simulink model "POWER_SYSTEM_FULL"  (R2025a)
settings: Solver=ode23t  StartTime=0  StopTime=5  FixedStep=1e-06  MinStep=1e-06  AbsTol=1e-6
model workspace (MAT data in the model file):
  CONTROL_INI : object (value not decoded)
  MODEL_INI : object (value not decoded)
  initialMemoryState = [1.15301991484 1.15301991484 1.15301991484 1.15301991484 0.612188611368 0.612188611368 0.612188611368 0.612188611368 -1.07438763375 -1.07438763375 -1.0821166602 -1.0821166602 ... (40 elements, 40x1)]
symbols that are objects in the model workspace (value not decoded): CONTROL_INI, MODEL_INI
undefined symbols (not defined in the file or in its folder): CONTROL, MODEL, monitorDFIG, pref_mask_vec, qref_mask_vec
(part 2 of 3)

== matlab function POWER_SYSTEM_FULL/DFIG ==
  settings: updateMethod=CONTINUOUS  sampleTime=MODEL_INI.PARAM.SIM_SAMPLING_TIME
  data: STATE input; INPUT input size=4*MODEL_INI.DFIG.PARAM.nDFIG+3; MODEL_IN input Bus: MODEL_Bus; STATE_DERIVATIVE output; OUTPUT output size=10*MODEL_INI.DFIG.PARAM.nDFIG; MODEL output Bus: MODEL_Bus; outSignals output; breaker_status input size=[1,4]; vw_delta input size=[1,4]
function [STATE_DERIVATIVE,OUTPUT,MODEL,outSignals] = DFIG_MODEL(STATE,INPUT,MODEL_IN,breaker_status, vw_delta)

%% COPY MODEL_BUS
MODEL = MODEL_IN;
nDFIG = 4;

%--------------------------------------------------------------------------
%% PARAMETERS
%--------------------------------------------------------------------------
% Rated frequency
f0 = MODEL.BASE.f0;
w0 = 2*pi*f0;
%--------------------------------------------------------------------------
% Induction machine parameters
%--------------------------------------------------------------------------
% Magnetizing reactance
Lm = MODEL.DFIG.PARAM.Lm_pu;
% Stator and rotor leakage reactances
ls = MODEL.DFIG.PARAM.Lsig_s_pu;
lr = MODEL.DFIG.PARAM.Lsig_r_pu;
% Stator and rotor resistances
Rs = MODEL.DFIG.PARAM.Rs_pu;
Rr = MODEL.DFIG.PARAM.Rr_pu;
% Auxiliar electric parameters
Ls = Lm + ls;
Lr = Lm + lr;
sg = 1 - Lm.^2./Ls./Lr;
%--------------------------------------------------------------------------
% DC-link
%--------------------------------------------------------------------------
% DC-link capacitor
Cdc = MODEL.DFIG.PARAM.Cdc_pu;
%--------------------------------------------------------------------------
% DC-LINK BRAKING CHOPPER  (Reviewer 1, point 2 -- fault ride-through)
%--------------------------------------------------------------------------
% LOCAL CONSTANTS, deliberately NOT read from the MODEL bus: adding a bus
% field would change the bus definition and force bus regeneration, which
% project_config.json classifies as a dangerous structural modification.
% Same convention as the converter current limiter in the CONTROL chart.
%
% WHY IT EXISTS -- measured, not speculative.  With the converter current
% limiter armed, a deep sag drove Vdc to 1.52 pu.  Without a chopper the
% DFIG has no way to dump rotor power when the GSC cannot export it: during
% a sag the terminal voltage collapses, the GSC's exportable power falls to
% ~0, and the rotor keeps delivering into the DC link.  No fault-ride-through
% claim is credible without it.
%
% CHOP_EN  Master enable.  0 = DISABLED (default), 1 = ARMED.  With
%          CHOP_EN = 0 the dissipation term is multiplied out to exactly
%          zero, so the model reproduces the no-chopper behaviour bit-for-bit
%          and every published result is unchanged.
CHOP_EN = 0;
%
% VDC_CHOP_ON / VDC_CHOP_OFF  Engage / release thresholds [pu on
%          MODEL.DFIG.BASE.Udc_base = 1200 V], against Vdc_ref = 1.0 pu.
%            VDC_CHOP_OFF = 1.05 pu = 1260 V  -- fully released below this.
%            VDC_CHOP_ON  = 1.10 pu = 1320 V  -- engage threshold.
%          1.05 pu leaves 5 % headroom above nominal so that normal operation
%          and normal transients never reach the chopper.  1.10 pu engages
%          well below the ~1.15-1.20 pu region where DC-link over-voltage
%          protection would trip a real converter, so the chopper acts BEFORE
%          the trip rather than instead of it.  The 0.05 pu band is the
%          conventional "few percent" hysteresis width.
%
%          THEIR ROLE IN THE DUTY REGULATOR (see K_CHOP below): VDC_CHOP_ON is
%          the REGULATION SETPOINT the duty drives Vdc toward, and the band
%          VDC_CHOP_ON - VDC_CHOP_OFF = 0.05 pu is the regulator's DROOP, i.e.
%          the reciprocal of its proportional gain.  Both constants keep their
%          numerical values and their engineering meaning; what changed is that
%          the chopper now MODULATES around VDC_CHOP_ON instead of being pinned
%          at full duty from VDC_CHOP_ON upwards.
VDC_CHOP_ON  = 1.10;
VDC_CHOP_OFF = 1.05;
%
% R_CHOP   Braking-resistor value [pu on MODEL.DFIG.BASE.Zdc_base =
%          Udc_base^2/Sb = 1200^2/2.1034e6 = 0.684605 ohm].
%
%          SIZING -- absorb the rotor power at the worst condition:
%            1. Measured at the optimisation operating point (from the stored
%               LIN_MODEL_VI_OPT): wr = 1.1575, so slip s = 1 - wr = -0.1575
%               (super-synchronous), stator power Ps = 0.849 pu, giving
%               rotor power |Pr| = |s|*Ps = 0.1337 pu flowing OUT of the
%               rotor and into the DC link.
%            2. Worst case: during the sag the rotor ACCELERATES (the slow
%               rotor-speed runaway already characterised), so |s| grows from
%               0.1575 toward the converter's design slip limit of 0.30.  At
%               |s| = 0.30 with stator power at rated 1.0 pu, |Pr| = 0.30 pu.
%            3. The GSC cannot help: at 0.05 pu retained voltage, clamped to
%               its 0.34 pu current rating, its exportable power is only
%               0.34*0.05 = 0.017 pu ~ 0.  So essentially ALL of Pr must be
%               dissipated by the chopper.
%            4. Design margin x1.67 over 0.30 pu to cover the rotor-current
%               surge at fault inception, where the instantaneous P_RSC is
%               well above the steady-state rotor power:
%                     P_chop_rated = 0.50 pu  (= 1.05 MW at Sb = 2.1034 MVA)
%            5. The resistor was sized so that the ORIGINAL on/off law reached
%               full dissipation at Vdc = VDC_CHOP_ON:
%                     R_CHOP = VDC_CHOP_ON^2 / P_chop_rated
%                            = 1.10^2 / 0.50 = 1.21 / 0.50 = 2.42 pu
%               Physical value: 2.42 * 0.684605 = 1.6567 ohm.
%          CROSS-CHECK in SI: at 1320 V across 1.6567 ohm the resistor
%          dissipates 1320^2/1.6567 = 1.0517 MW = 0.500 pu of 2.1034 MVA.
%
%          R_CHOP IS UNCHANGED BY THE MOVE TO A REGULATING DUTY.  It is the
%          resistor's MAXIMUM CAPABILITY, reached only at duty 1; what the duty
%          regulator changes is HOW MUCH OF THAT CAPABILITY IS USED.  Under the
%          regulator (see K_CHOP) duty 1 is reached at 1.15 pu rather than at
%          1.10 pu, where the same resistor dissipates 1.15^2/2.42 = 0.5465 pu
%          -- a 9.3 % increase in peak capability, which is inside the x1.67
%          design margin of step 4 and does not re-open the sizing.
R_CHOP = 2.42;
%
% K_CHOP   Proportional gain of the chopper DUTY REGULATOR
%          [pu duty per pu DC-link voltage].
%
%          WHY THE ON/OFF LAW WAS WRONG -- MEASURED, not speculative.  The
%          first implementation set the duty from the position of Vdc inside
%          the threshold band and SATURATED it at 1 from VDC_CHOP_ON upwards.
%          That makes the chopper a BANG-BANG FULL-POWER DRAIN the moment it is
%          armed.  In the deep-sag run (retained 0.05 pu, SCR = 1, P = 0.8) it
%          dissipated Vdc^2/R_CHOP = 1.23^2/2.42 = 0.625 pu at Vdc = 1.23 pu
%          against an actual DC-link surplus of order 0.1-0.2 pu, and over the
%          peak-to-zero window its time-weighted mean P_CHOP = +0.2885 pu was
%          the LARGEST drain term in the balance -- larger than the GSC export.
%          The chopper installed to protect the DC link was a material
%          contributor to the collapse it was meant to prevent, and Vdc went on
%          to reverse sign to -0.6123 pu.
%
%          WHY IT WAS THE WRONG AVERAGE.  A hysteretic chopper does not hold
%          its IGBT on: it CYCLES it, and the MEAN duty over a switching period
%          is whatever the DC-link power balance demands -- it is not a
%          function of where Vdc happens to sit.  In an AVERAGED converter
%          model Vdc is a slow state, not a fast carrier, so the faithful
%          average of that cycling is a REGULATOR: a duty that closes a loop
%          around Vdc and therefore dissipates the SURPLUS, which is exactly
%          what the switching hardware achieves.  A static band-position ->
%          duty map is not the average of a hysteretic chopper; it is the
%          average of a chopper whose IGBT is stuck on.
%
%          THE LAW -- proportional on the over-voltage, referenced to the
%          ENGAGE threshold, saturated to [0,1] and STILL PURELY ALGEBRAIC
%          (no new states, no bus fields):
%                 d_chop = sat( K_CHOP*(Vdc - VDC_CHOP_ON), 0, 1 )
%
%          THE GAIN, and why this value:
%                 K_CHOP = 1/(VDC_CHOP_ON - VDC_CHOP_OFF) = 1/0.05 = 20
%          It is the reciprocal of the EXISTING threshold band, so no new
%          constant is introduced and the two thresholds keep exact meanings
%          (setpoint and droop).  Three consequences, and they are the
%          justification:
%            1. STEADY-STATE ACCURACY.  The droop is 1/K_CHOP = 0.05 pu, so for
%               any surplus within the resistor's capability the chopper holds
%               Vdc inside [1.10, 1.15] pu and the dissipated power settles at
%               the SURPLUS, not at the rating.  Worked against the measured
%               number above: at a 0.12 pu surplus the loop settles at
%               d = 0.12*2.42/1.11^2 = 0.236, burning 0.12 pu -- not 0.625 pu.
%            2. SOLVER STIFFNESS -- MEASURED, NOT ASSUMED.  A slope of 0 -> 1
%               over 0.05 pu is EXACTLY the slope the previous implementation
%               already carried, only shifted up by one band.  The closed-loop
%               DC-link mode it creates,
%                  lambda = -(w0/Cdc)*K_CHOP*(2*Vdc - VDC_CHOP_ON)/R_CHOP
%                         ~ -5.9e3 rad/s   (tau ~ 0.17 ms at Vdc ~ 1.10),
%               is therefore the SAME mode that the 50 % and the 20 % sag cases
%               already integrated to completion under ode23t with MaxStep 1e-3
%               and MinStep 1e-6.  This change introduces NO new fast mode.  A
%               stiffer gain (K_CHOP = 100 would hold Vdc within 1 %) was
%               rejected for exactly that reason: it would put a 34 us mode
%               into a model that has already been observed to fail Newton
%               convergence at hmin in this operating region.
%            3. SATURATION POINT.  Full duty falls at VDC_CHOP_ON + 1/K_CHOP =
%               1.15 pu -- the bottom of the 1.15-1.20 pu band where a real
%               converter's DC-link over-voltage protection trips.  So the
%               resistor reaches its rated dissipation exactly where a real
%               machine would be about to trip, and modulates below it.  This
%               is the same "act BEFORE the trip" intent already recorded for
%               the thresholds, now expressed in the duty rather than in R.
%
%          WHAT THIS DOES NOT CLAIM.  Above 1.15 pu the duty IS 1 and the
%          resistor DOES dissipate its full capability.  That is not a
%          modelling artefact -- a real hysteretic chopper at 1.23 pu is also
%          hard on, continuously.  What is fixed here is the pinning of the
%          duty at 1 across the WHOLE armed range; what no duty law can fix is
%          an over-sized resistor, and R_CHOP is deliberately left at its
%          original value so that this change is the duty and nothing else.
K_CHOP = 1./(VDC_CHOP_ON - VDC_CHOP_OFF);
%--------------------------------------------------------------------------
% DC-LINK DIVISION GUARD -- NUMERICAL, UNCONDITIONAL
%--------------------------------------------------------------------------
% VDC_FLOOR  Denominator floor for the DC-link current map  idc = Pdc/Vdc.
%          This is a NUMERICAL GUARD, NOT a control or protection feature, so
%          it is DELIBERATELY NOT gated on CHOP_EN or on any other switch: an
%          unguarded division belongs in no version of the model.  It is the
%          exact analogue of VS_FLOOR in the CONTROL chart, one chart over.
%
%          WHY IT EXISTS -- measured, not speculative.  In a deep sag (0.05 pu
%          retained) the DC link does NOT over-charge, it DRAINS: the terminal
%          voltage collapses, so the GSC can import at most 0.34*0.05 = 0.017
%          pu while the RSC keeps drawing from the capacitor.  Vdc was measured
%          falling through 0.3219 pu at the instant the solver died with
%          NewtonIterationFailure at hmin, 8.68 ms after inception.  As
%          Vdc -> 0 both the map idc = Pdc/Vdc and its Jacobian entry
%          d(idc)/d(Vdc) = -Pdc/Vdc^2 blow up, and nothing downstream can
%          rescue it: min/max propagate Inf and NaN rather than clamping them.
%          The braking chopper cannot help -- it only acts above
%          VDC_CHOP_OFF = 1.05 pu and addresses the OPPOSITE excursion.
%
%          VALUE: 0.50 pu = 600 V on Udc_base = 1200 V.  The justification is
%          that at and below this DC voltage the RSC has already lost control
%          authority, so the AVERAGED converter model -- whose core assumption
%          is that vr and vg are imposed EXACTLY as commanded -- is outside its
%          validity range regardless of what the division does:
%            - With SVPWM a two-level bridge synthesises at most Vdc/sqrt(2)
%              of line-to-line RMS AC voltage.  At Vdc = 0.50 pu = 600 V that
%              is 424.3 V, i.e. 424.3/2070 = 0.205 pu on the rotor base
%              (Ur_open_rotor_V = 2070 V = 3 pu of Ub = 690 V).
%            - The rotor back-EMF ALONE is |s|*|Fs|*Lm/Ls = 0.1575*1*
%              2.0033/2.0731 = 0.152 pu at the pre-fault slip, and it GROWS as
%              the rotor accelerates during the fault.  So at 0.50 pu the RSC
%              retains under 35 % margin over the back-EMF BEFORE the resistive
%              and di/dt terms -- it can no longer impose the commanded rotor
%              voltage, and the model has stopped describing the machine.
%            - For scale, the DC link is sized for the full +-0.30 design slip:
%              |vr| = 0.30*2070 = 621 V needs Vdc >= sqrt(2)*621 = 878 V =
%              0.73 pu, against the 1.0 pu nominal.
%
%          The floor is INACTIVE in every legitimate transient measured.  The
%          deepest Vdc excursion in any run that integrates to completion is
%          0.6679 pu (50 % sag, 150 ms, limiter and chopper armed), 25 % above
%          the floor; the 20 % / 500 ms case reaches 0.6892 pu.  At both
%          linearisation operating points Vdc = 1.0 pu exactly, so
%          Vdc_safe == Vdc and the guard is invisible to the small-signal
%          model.  That is verified, not asserted, by the zero-difference
%          regression at all four switch combinations.
VDC_FLOOR = 0.50;
%--------------------------------------------------------------------------
% DC-LINK DIODE CLAMP -- PHYSICS, UNCONDITIONAL, NO NEW STATES
%--------------------------------------------------------------------------
% VDC_DIODE / VDC_DIODE_BAND  One-sided LOWER clamp on the DC-link voltage,
%          enforcing in the averaged model what the converters' ANTI-PARALLEL
%          DIODES enforce in hardware: the DC link cannot be discharged
%          through zero.  Measured motivation -- in a deep sag the stator
%          power collapses, there is no slip power left to trap, P_RSC FLIPS
%          POSITIVE (it pushes INTO the rotor to hold |ir| at the limit
%          against collapsed flux) while the GSC still exports, and the link
%          drains to Vdc = -0.5825 pu.  A negative DC-link voltage is not a
%          small error, it is impossible: the diodes clamp it.
%
%          THIS IS NOT VDC_FLOOR AND MUST NOT BE CONFLATED WITH IT.  They are
%          different objects doing different jobs and the paper must keep them
%          apart:
%            - VDC_FLOOR = 0.50 pu is a NUMERICAL guard on a DIVISION.  It
%              bounds the DENOMINATOR of idc = Pdc/Vdc so the map and its
%              Jacobian stay finite.  It is a statement about ARITHMETIC.
%              Where it is active the trajectory is an ARTEFACT OF THE GUARD
%              and no quantitative claim may rest on it.
%            - VDC_DIODE is a PHYSICAL constraint on the STATE.  It says a
%              capacitor bridged by anti-parallel diodes cannot reverse
%              polarity.  Where it is active the trajectory is STILL PHYSICS:
%              it is the physics of a link being held up by its own diodes.
%          A run that touches VDC_FLOOR has left the model's validity range;
%          a run that touches VDC_DIODE has not.  Reporting the two as the
%          same event would overstate the model's reach in exactly the way
%          quoting the source voltage instead of the PCC voltage does.
%
%          WHY IT CANNOT BE A max() ON Vdc.  Vdc is STATE 6, not an algebraic
%          quantity.  A max() here would clamp the value the chart READS while
%          the integrator went on driving the true state further negative; the
%          clamp would then silently unlatch on the way back up, and the
%          reported Vdc would no longer be the model's own state.  The
%          physically correct statement is a ONE-SIDED CONSTRAINT ON THE
%          DERIVATIVE: discharge is progressively refused as Vdc approaches
%          the clamp, charge is never impeded.  That is what is implemented at
%          the dVdc assignment below, and it adds NO state and NO bus field.
%
%          VALUE: 0.05 pu = 60 V on Udc_base = 1200 V.  Zero is the strict
%          physical bound; 0.05 pu sits just above it, deliberately.  First,
%          it keeps the state away from the exact zero at which the UNGUARDED
%          map idc = Pdc/Vdc changes sign, so the diode clamp does not lean on
%          VDC_FLOOR to stay finite and the two stay independent -- which is
%          the whole point of separating them.  Second, a real diode clamp
%          holds the link at the RECTIFIED PEAK of the AC side, which is well
%          above zero; 0.05 pu is a deliberately conservative stand-in for
%          that bound, not an attempt to model it.
%
%          SCOPE, STATED PLAINLY: the entire clamp lives at 0.15 pu and below,
%          i.e. wholly INSIDE the region VDC_FLOOR has already declared
%          numerically guarded.  It can therefore only ever rescue criterion
%          (a) (Vdc > 0) and CANNOT move criterion (b) (Vdc >= VDC_FLOOR).
%          It is not intended to.  Moving (b) is the RSC blocking's job, one
%          chart over -- the clamp bounds the consequence, the blocking
%          removes the cause.
VDC_DIODE = 0.05;
% VDC_DIODE_BAND  Blend width [pu] of the clamp gate.
%          A HARD kink at the clamp would be worse than the singularity it
%          replaces: it makes dVdc discontinuous in a state and forces ode23t
%          to chatter its Newton iteration across the crossing.  The gate is
%          therefore a SMOOTHSTEP s^2*(3-2s) over [VDC_DIODE, VDC_DIODE+BAND],
%          which is C1 -- ZERO SLOPE AT BOTH ENDS.
%            - Zero slope at the UPPER end is what makes the clamp exactly
%              invisible to the linearisation.  The gate is not merely EQUAL
%              to 1 at the operating point (Vdc = 1.0 pu, 8.5 band-widths
%              above the top of the band); its derivative with respect to Vdc
%              is also exactly 0 there, so no numericalpert step of order
%              1e-5 can see it.
%            - Zero slope at the LOWER end gives a soft landing: the approach
%              to the clamp decelerates quadratically rather than stopping in
%              a corner, so the solver is not asked to resolve an impact.
VDC_DIODE_BAND = 0.10;
%--------------------------------------------------------------------------
% GSC filter
%--------------------------------------------------------------------------
% GSC filter resistance
Rfg = MODEL.DFIG.PARAM.Rfgsc_pu;
% GSC filter reactance
Lfg = MODEL.DFIG.PARAM.Lfgsc_pu;
%--------------------------------------------------------------------------
% Transformer
%--------------------------------------------------------------------------
% Transformer resistance
Rt = MODEL.DFIG.PARAM.Rt_pu;
% Transformer inductance
Lt = MODEL.DFIG.PARAM.Lt_pu;
%--------------------------------------------------------------------------
% Mechanical model (2 masses)
%--------------------------------------------------------------------------
Ht = MODEL.DFIG.PARAM.Ht_pu;
Dt = MODEL.DFIG.PARAM.Dt_pu;
Hg = MODEL.DFIG.PARAM.Hg_pu;
Dg = MODEL.DFIG.PARAM.Dg_pu;
Dtg = MODEL.DFIG.PARAM.Dtg_pu;
Ktg = MODEL.DFIG.PARAM.Ktg_pu;
%--------------------------------------------------------------------------
% Turbine
%--------------------------------------------------------------------------
% Turbine data
turbineData = MODEL.DFIG.PARAM.turbineData;

%--------------------------------------------------------------------------
% State-space representation with transformer
%--------------------------------------------------------------------------
% it = -(ig + is)
% 1/w0*dFs + 1j*w*Fs         = vs - Rs.*is;       % is flows into the IM 
% 1/w0*dFr + 1j*(w - wr).*Fr = vr - Rr.*ir;       % ir flows into the IM
% 1/w0*dFg + 1j*w*Fg         = vs - vg - Rfg.*ig; % ig flows into the GSC
% 1/w0*dFt + 1j*w*Ft         = vs - vp - Rt.*it;  % it flows into the PCC
%--------------------------------------------------------------------------
% Fst = Fs - Ft
% Fgt = Fg - Ft
%--------------------------------------------------------------------------
% 1./w0.*dFst + 1j*w.*Fst = vp + Rt.*it - Rs.*is;
% 1./w0.*dFgt + 1j*w.*Fgt = vp + Rt.*it - vg - Rfg.*ig;
%--------------------------------------------------------------------------
% 1./w0.*dFst + 1j*w.*Fst = vp - (Rs + Rt).*is - Rt.*ig;
% 1./w0.*dFgt + 1j*w.*Fgt = vp - vg - Rt.*is - (Rfg + Rt).*ig;
%--------------------------------------------------------------------------
% Fg = Lfg.*ig
% Ft = Lt.*it
% Fs = Ls.*is + Lm.*ir
% Fr = Lm.*is + Lr.*ir
%--------------------------------------------------------------------------
% Fgt = Lfg.*ig - Lt.*it = (Lfg + Lt).*ig + Lt.*is
% Fst = Ls.*is + Lm.*ir - Lt.*it = (Ls + Lt).*is + Lt.*ig + Lm.*ir
% Lm.*ir = Lm./Lr.*(Fr - Lm.*is)
% Fst - Lm./Lr.*Fr = (sg.*Ls + Lt).*is + Lt.*ig
%--------------------------------------------------------------------------
% [Fgt ; Fst - Lm./Lr.*Fr] = [Lfg+Lt   Lt ; Lt  sg*Ls+Lt]*[ig ; is]
% [ig ; is] = inv([Lfg+Lt   Lt ; Lt  sg*Ls+Lt])*[Fgt ; Fst - Lm./Lr.*Fr]
% |Lfg+Lt   Lt ; Lt  sg*Ls+Lt| = (Lfg+Lt)*(sg*Ls+Lt) - Lt^2 = 
%                             = sg*Ls*Lfg + (Lfg+sg*Ls)*Lt
% inv([Lfg+Lt   Lt ; Lt  sg*Ls+Lt]) = [sg*Ls+Lt -Lt ; -Lt Lfg+Lt]/(sg*Ls*Lfg + (Lfg+sg*Ls)*Lt)
%--------------------------------------------------------------------------
% ig = ((sg.*Ls+Lt).*Fgt - Lt.*(Fst - Lm./Lr.*Fr))./(sg.*Ls.*Lfg + (Lfg+sg*Ls).*Lt)
% is = (-Lt.*Fgt  + (Lfg + Lt).*(Fst - Lm./Lr.*Fr))./(sg.*Ls.*Lfg + (Lfg+sg*Ls).*Lt)
% it = -(ig + is)
% Fs = Ls.*is + Lm.*ir = Ls.*is + Lm./Lr.*(Fr - Lm.*is) = sg.*Ls.*is + Lm./Lr.*Fr;
% Ft = Fs - Fst;
% Fg = Fgt + Ft;
% ir = 1./Lm.*(Fs - Ls.*is)
% dis = (-Lt.*Fgt  + (Lfg + Lt).*(dFst - Lm./Lr.*dFr))./(sg.*Ls.*Lfg + (Lfg+sg*Ls).*Lt)
% 1./w0*dFs = sg.*Ls.*dis + Lm./Lr.*dFr
% vs = 1/w0*dFs + 1j*w*Fs + Rs*is
%--------------------------------------------------------------------------

%--------------------------------------------------------------------------
%% STATE
%--------------------------------------------------------------------------
% Stator flux - Transformer flux
%--------------------------------------------------------------------------
Fst_r = STATE(1,:);
Fst_i = STATE(2,:);
Fst = Fst_r + 1j*Fst_i;
%--------------------------------------------------------------------------
% Rotor flux
%--------------------------------------------------------------------------
Fr_r = STATE(3,:);
Fr_i = STATE(4,:);
Fr = Fr_r + 1j*Fr_i;
%--------------------------------------------------------------------------
% Rotor speed
%--------------------------------------------------------------------------
wr = STATE(5,:);
%--------------------------------------------------------------------------
% DC-Link voltage
%--------------------------------------------------------------------------
Vdc = STATE(6,:);
%--------------------------------------------------------------------------
% GSC flux - transformer flux
%--------------------------------------------------------------------------
Fgt_r = STATE(7,:);
Fgt_i = STATE(8,:);
Fgt = Fgt_r + 1j*Fgt_i;
%--------------------------------------------------------------------------
% Mechanical shaft
%--------------------------------------------------------------------------
wt = STATE(9,:);
Ttg = STATE(10,:);

%--------------------------------------------------------------------------
%% INPUT
%--------------------------------------------------------------------------
% INPUT = [vrr ; vri ; vgr ; vgi ; w ; vpr ; vpi]
nDFIG = 4;
vrr = INPUT(0*nDFIG + (1:nDFIG))';
vri = INPUT(1*nDFIG + (1:nDFIG))';
vgr = INPUT(2*nDFIG + (1:nDFIG))';
vgi = INPUT(3*nDFIG + (1:nDFIG))';
w   = INPUT(4*nDFIG + 1);
vpr = INPUT(4*nDFIG + 2);
vpi = INPUT(4*nDFIG + 3);
%--------------------------------------------------------------------------
% RSC voltage
%--------------------------------------------------------------------------
MODEL.DFIG.INPUT.vRSC_r = vrr;
MODEL.DFIG.INPUT.vRSC_i = vri;
vr = vrr + 1j*vri;
%--------------------------------------------------------------------------
% GSC voltage
%--------------------------------------------------------------------------
MODEL.DFIG.INPUT.vGSC_r = vgr;
MODEL.DFIG.INPUT.vGSC_i = vgi; 
vg = vgr + 1j*vgi;
%--------------------------------------------------------------------------
% PCC voltage
%--------------------------------------------------------------------------
MODEL.DFIG.INPUT.vPCC_r = vpr*ones(1,nDFIG);
MODEL.DFIG.INPUT.vPCC_i = vpi*ones(1,nDFIG); 
vp = vpr + 1j*vpi;
%--------------------------------------------------------------------------
% Grid frequency [pu]
%--------------------------------------------------------------------------
MODEL.GRID.OUTPUT.f_pu = w;
%--------------------------------------------------------------------------
% Wind speed [m/s]
%--------------------------------------------------------------------------
windSpeed = MODEL.DFIG.INPUT.windSpeed + vw_delta;
%% vw_delta [1x4]: additive wind speed perturbation (m/s), zeros at op point
%--------------------------------------------------------------------------
% Turbine pitch [deg]
%--------------------------------------------------------------------------
pitch = MODEL.DFIG.INPUT.turbinePitch;


%--------------------------------------------------------------------------
%% ELECTRIC VARIABLES
%--------------------------------------------------------------------------
% Stator current
%--------------------------------------------------------------------------
is = (-Lt.*Fgt + (Lfg + Lt).*(Fst - Lm./Lr.*Fr))./(sg.*Ls.*Lfg + (Lfg+sg.*Ls).*Lt);
isr = real(is);
isi = imag(is);
%--------------------------------------------------------------------------
% Fluxes
%--------------------------------------------------------------------------
Fs = sg.*Ls.*is + Lm./Lr.*Fr;
Ft = Fs - Fst;
Fg = Fgt + Ft;
%--------------------------------------------------------------------------
% Rotor current
%--------------------------------------------------------------------------
ir = 1./Lm.*(Fs - Ls.*is);
irr = real(ir);
iri = imag(ir);
%--------------------------------------------------------------------------
% Grid current
%--------------------------------------------------------------------------
ig = 1./Lfg.*Fg; 
igr = real(ig); 
igi = imag(ig);
%--------------------------------------------------------------------------
% Transformer current
%--------------------------------------------------------------------------
it = 1./Lt.*Ft; 
itr = real(it); 
iti = imag(it);
%--------------------------------------------------------------------------
% Electric torque (motor torque)
%--------------------------------------------------------------------------
% Te = imag(is*conj(Fs))/sqrt(3)
% Fs = Ls*is + Lm*ir
% Te = imag(is*conj(Ls*is + Lm*ir))/sqrt(3) = Lm*imag(is*conj(ir))/sqrt(3)
Te = Lm.*imag(is.*conj(ir))/sqrt(3);
%--------------------------------------------------------------------------
% Power computation in DC link
%--------------------------------------------------------------------------
P_GSC = real(vg.*conj(ig))/sqrt(3);
P_RSC = real(vr.*conj(ir))/sqrt(3);
Pdc = P_GSC - P_RSC;
%--------------------------------------------------------------------------
% DC-link braking chopper -- CONDITIONAL DISSIPATION, PURELY ALGEBRAIC
%--------------------------------------------------------------------------
% Sign convention check: Pdc = P_GSC - P_RSC charges the capacitor, since
% dVdc = w0*idc/Cdc with idc = Pdc/Vdc.  Super-synchronously P_RSC < 0 (the
% rotor DELIVERS), and during a sag P_GSC -> 0 while P_RSC stays negative, so
% Pdc > 0 and Vdc rises.  The chopper therefore SUBTRACTS from Pdc.
%
% d_chop is the chopper DUTY CYCLE: the AVERAGED-MODEL representation of a
% hysteresis-cycled chopper, written as a PROPORTIONAL REGULATOR on the
% DC-link over-voltage.  A true two-valued relay with engage/release memory is
% by definition STATEFUL and the constraint here is NO NEW STATES; but the
% averaged duty is not merely a workaround for that constraint, it is the
% CORRECT representation, because the quantity a real chopper's switching
% produces on the time scale this model resolves IS a mean duty.
%
% The mean duty of a hysteresis-cycled IGBT is set by the DC-LINK POWER
% BALANCE -- the chopper cycles at whatever ratio dissipates the instantaneous
% surplus and thereby holds Vdc at its threshold.  It is NOT a static function
% of where Vdc sits.  Mapping band position directly onto duty (the previous
% implementation) pins the duty at 1 the moment Vdc leaves the band upwards,
% i.e. it averages a chopper whose IGBT is STUCK ON, and it dumps the
% resistor's full capability whenever armed rather than the surplus.  That was
% measured to be the largest single drain term in the deep-sag DC-link
% collapse (see the K_CHOP block above for the numbers).
%
% The regulator form fixes exactly that: VDC_CHOP_ON is the SETPOINT the loop
% drives Vdc toward, K_CHOP = 1/(VDC_CHOP_ON - VDC_CHOP_OFF) is the droop, and
% the saturation to [0,1] is the physical duty limit.  It is still continuous,
% so it does not chatter the variable-step solver the way a bare relay would,
% and it is still purely algebraic.
d_chop = min(max(K_CHOP.*(Vdc - VDC_CHOP_ON),0),1);
% Dissipated power [pu].  Identically 0 when CHOP_EN = 0, and ALSO identically
% 0 whenever Vdc <= VDC_CHOP_ON regardless of CHOP_EN -- which is why the
% linearisation at the operating point (Vdc = 1.0 pu) is unaffected in both
% switch states: the clamp is FLAT there, so the term and its derivative with
% respect to every state are exactly zero.  The margin from the operating
% point to the start of the ramp is now 0.10 pu rather than 0.05 pu, i.e.
% TWICE the previous distance, against a numericalpert step of order 1e-5.
P_CHOP = CHOP_EN .* d_chop .* Vdc.^2 ./ R_CHOP;
Pdc = Pdc - P_CHOP;
%--------------------------------------------------------------------------
% Current in DC link
%--------------------------------------------------------------------------
% Guarded denominator -- see VDC_FLOOR above.  A single unconditional max() is
% sufficient and is NOT gated on any switch.  It also fixes the SIGN: an
% unguarded 1/Vdc flips sign if a solver trial iterate drives Vdc through zero,
% which no Newton iteration can recover from.  Below the floor the map is flat
% in Vdc, so the Jacobian entry -Pdc/Vdc^2 is replaced by exactly 0 instead of
% diverging.  Vdc itself, not Vdc_safe, is what leaves the chart as OUTPUT and
% feeds the chopper duty and the CONTROL chart, so the guard changes the
% DERIVATIVE map only and never falsifies a reported quantity.
Vdc_safe = max(Vdc, VDC_FLOOR);
idc = Pdc./Vdc_safe;

%--------------------------------------------------------------------------
%% MECHANICAL VARIABLES
%--------------------------------------------------------------------------
% Turbine mechanical power
%--------------------------------------------------------------------------
% Mechanical power = 1/2*Cp(Lambda,Pitch)*ro*pi*R^2*windSpeed^3
Pm = WIND_TURBINE_OP(pitch,windSpeed,wt,turbineData);
Pm = Pm.*(Pm>0);
%--------------------------------------------------------------------------
% Turbine mechanical torque
%--------------------------------------------------------------------------
Tm = Pm./wt;

%--------------------------------------------------------------------------
%% STATE DERIVATIVE
%--------------------------------------------------------------------------
% Stator - Transformer Flux 
%--------------------------------------------------------------------------
% 1./w0.*dFst + 1j*w.*Fst = vp - (Rs + Rt).*is - Rt.*ig;
dFst = w0.*(vp - Rt.*ig - (Rt + Rs).*is - 1j.*w.*Fst);
dFst_r = real(dFst); 
dFst_i = imag(dFst);
%--------------------------------------------------------------------------
% Rotor Flux
%--------------------------------------------------------------------------
dFr = w0.*(vr - Rr.*ir - 1j.*(w - wr).*Fr);
dFr_r = real(dFr); 
dFr_i = imag(dFr);
%--------------------------------------------------------------------------
% DC-Link voltage
%--------------------------------------------------------------------------
% DIODE CLAMP -- one-sided constraint on the DERIVATIVE (see VDC_DIODE above).
% Charging is never impeded; discharging is faded out as Vdc approaches the
% clamp level.  The split
%       dVdc = max(dVdc_raw,0) + g.*min(dVdc_raw,0)
% is an EXACT IDENTITY when g = 1, because max(x,0) + min(x,0) == x for every
% x -- in floating point as well as in algebra, since one term is always
% exactly x and the other exactly 0.  Above the band the derivative is
% therefore bit-for-bit the unclamped one, which is why the small-signal
% regression stays EXACTLY zero rather than merely small.
dVdc_raw = w0.*idc./Cdc;
s_diode  = min(max((Vdc - VDC_DIODE)./VDC_DIODE_BAND, 0), 1);
g_diode  = s_diode.^2.*(3 - 2.*s_diode);
dVdc     = max(dVdc_raw,0) + g_diode.*min(dVdc_raw,0);
%--------------------------------------------------------------------------
% GSC - Transformer Flux
%--------------------------------------------------------------------------
% 1./w0.*dFgt + 1j*w.*Fgt = vp - vg - Rt.*is - (Rfg + Rt).*ig;
dFgt = w0.*(vp - vg - Rt.*is - (Rt + Rfg).*ig - 1j*w.*Fgt);
dFgt_r = real(dFgt); 
dFgt_i = imag(dFgt);
%--------------------------------------------------------------------------
% Turbine and shaft dynamics
%--------------------------------------------------------------------------
dwt = (1/2)./Ht.*(Tm - Dt.*wt - Ttg - Dtg.*(wt-wr));
dTtg = w0*Ktg.*(wt-wr);
% dTtg = Ktg.*(wt-wr);
dwr = (1/2)./Hg.*(Ttg + Te - Dg.*wr + Dtg.*(wt-wr));
%--------------------------------------------------------------------------
% State derivative
%--------------------------------------------------------------------------
STATE_DERIVATIVE = [dFst_r ; dFst_i ; dFr_r ; dFr_i ; dwr ; ....
    dVdc ; dFgt_r ; dFgt_i ; dwt ; dTtg];

%--------------------------------------------------------------------------
% BREAKER LOGIC: freeze states of disconnected generators
%--------------------------------------------------------------------------
STATE_DERIVATIVE = STATE_DERIVATIVE .* breaker_status;

%--------------------------------------------------------------------------
%% OUTPUT AND MEASURED VARIABLES
%--------------------------------------------------------------------------
% Stator voltage
%--------------------------------------------------------------------------
dis = (-Lt.*Fgt  + (Lfg + Lt).*(dFst - Lm./Lr.*dFr))./(sg.*Ls.*Lfg + (Lfg+sg.*Ls).*Lt);
dFs = sg.*Ls.*dis + Lm./Lr.*dFr;
vs = 1/w0*dFs + 1j*w*Fs + Rs.*is;
MODEL.DFIG.OUTPUT.vs_r = real(vs);
MODEL.DFIG.OUTPUT.vs_i = imag(vs);
%--------------------------------------------------------------------------
% Currents
%--------------------------------------------------------------------------
% Stator current into the IM
MODEL.DFIG.OUTPUT.is_r = isr;
MODEL.DFIG.OUTPUT.is_i = isi;
% Rotor current into the IM and from the RSC
MODEL.DFIG.OUTPUT.ir_r = irr;
MODEL.DFIG.OUTPUT.ir_i = iri;
% GSC current into the GSC
MODEL.DFIG.OUTPUT.ig_r = igr;
MODEL.DFIG.OUTPUT.ig_i = igi;
% Transformer current into the PCC and from the DFIG
MODEL.DFIG.OUTPUT.it_r = itr;
MODEL.DFIG.OUTPUT.it_i = iti;
%--------------------------------------------------------------------------
% DC-Link Voltage [pu]
%--------------------------------------------------------------------------
MODEL.DFIG.OUTPUT.Vdc = Vdc;
%--------------------------------------------------------------------------
% Converter and DC-Link powers
%--------------------------------------------------------------------------
MODEL.DFIG.OUTPUT.P_GSC = P_GSC;
MODEL.DFIG.OUTPUT.P_RSC = P_RSC;
MODEL.DFIG.OUTPUT.Pdc = Pdc;
%--------------------------------------------------------------------------
% Rotor speed [pu]
%--------------------------------------------------------------------------
MODEL.DFIG.OUTPUT.wr = wr;
%--------------------------------------------------------------------------
% Mechanical power [pu]
%--------------------------------------------------------------------------
MODEL.DFIG.OUTPUT.Pm = Pm;

%--------------------------------------------------------------------------
%% STATE UPDATE
%--------------------------------------------------------------------------
MODEL.DFIG.STATE = STATE;

%--------------------------------------------------------------------------
%% CONNECTIONS WITH THE POWER SYSTEM
%--------------------------------------------------------------------------
%--------------------------------------------------------------------------
% BREAKER LOGIC: zero currents of disconnected generators
%--------------------------------------------------------------------------
itr = itr .* breaker_status;
iti = iti .* breaker_status;
isr = isr .* breaker_status;
isi = isi .* breaker_status;
irr = irr .* breaker_status;
iri = iri .* breaker_status;
igr = igr .* breaker_status;
igi = igi .* breaker_status;

%--------------------------------------------------------------------------
% OUTPUT = [itr ; iti ; isr ; isi ; irr ; iri ; vsr ; vsi ; Vdc ; wr]
%--------------------------------------------------------------------------
OUTPUT = zeros(10*nDFIG,1);
OUTPUT(0*nDFIG + (1:nDFIG)) = itr(:);
OUTPUT(1*nDFIG + (1:nDFIG)) = iti(:);
OUTPUT(2*nDFIG + (1:nDFIG)) = isr(:);
OUTPUT(3*nDFIG + (1:nDFIG)) = isi(:);
OUTPUT(4*nDFIG + (1:nDFIG)) = irr(:);
OUTPUT(5*nDFIG + (1:nDFIG)) = iri(:);
OUTPUT(6*nDFIG + (1:nDFIG)) = real(vs(:));
OUTPUT(7*nDFIG + (1:nDFIG)) = imag(vs(:));
OUTPUT(8*nDFIG + (1:nDFIG)) = Vdc(:);
OUTPUT(9*nDFIG + (1:nDFIG)) = wr(:);

%% Output auxiliary signals
Sdfig = vs.*conj(it)/sqrt(3);
outSignals = [abs(vs(:)),real(Sdfig(:)),imag(Sdfig(:)),Vdc(:)];

return

== matlab function POWER_SYSTEM_FULL/LINE_GRID ==
  settings: updateMethod=CONTINUOUS  sampleTime=MODEL_INI.PARAM.SIM_SAMPLING_TIME
  data: STATE input; INPUT input size=2*MODEL_INI.DFIG.PARAM.nDFIG; MODEL_IN input Bus: MODEL_Bus; STATE_DERIVATIVE output; OUTPUT output size=3; MODEL output Bus: MODEL_Bus; il_r_IN input; il_i_IN input; f_OUT output; Vpcc_OUT output
function [STATE_DERIVATIVE,OUTPUT,MODEL,f_OUT,Vpcc_OUT] = LINE_GRID_MODEL(STATE,INPUT,MODEL_IN,il_r_IN,il_i_IN)

%% COPY MODEL_BUS
MODEL = MODEL_IN;
nDFIG = 4;

%--------------------------------------------------------------------------
%% PARAMETERS
%--------------------------------------------------------------------------
% Rated frequency
%--------------------------------------------------------------------------
f0 = MODEL.BASE.f0;
w0 = 2*pi*f0;

%--------------------------------------------------------------------------
% Grid resistence and inductance
%--------------------------------------------------------------------------
Rg = MODEL.GRID.PARAM.Rg_pu;
Lg = MODEL.GRID.PARAM.Lg_pu;
%--------------------------------------------------------------------------
% Node 1 resistance and capacitance
%--------------------------------------------------------------------------
Rn1 = MODEL.LINE.PARAM.Rn1_pu;
Cn1 = MODEL.LINE.PARAM.Cn1_pu;
%--------------------------------------------------------------------------
% Load perturbation injection node (1=PCC, 2=grid bus)
%--------------------------------------------------------------------------
load_node = MODEL.LINE.PARAM.load_node;
%--------------------------------------------------------------------------
% Speed governor
%--------------------------------------------------------------------------
% Damping (Deq_pu/2) and steady-state droop (2/Deq_pu)
Deq_pu = MODEL.GRID.PARAM.Deq_pu;
% Time constant [s]
Tgov = MODEL.GRID.PARAM.Tgov;
%--------------------------------------------------------------------------
% Turbine (second order: time constants Ttb1 and Ttb2
%--------------------------------------------------------------------------
% [(0.3*7) 1] / [(0.3*7) (0.3+7) 1]
% [(Ttb1*Ttb2) 1] / [(Ttb1*Ttb2) (Ttb1+Ttb2) 1]
% Time constants [s]
Ttb1 = MODEL.GRID.PARAM.Ttb1;
Ttb2 = MODEL.GRID.PARAM.Ttb2;
%--------------------------------------------------------------------------
% Grid inertia [s]
%--------------------------------------------------------------------------
H = MODEL.GRID.PARAM.H;

%--------------------------------------------------------------------------
%% STATE
%--------------------------------------------------------------------------
%--------------------------------------------------------------------------
% Speed governor (first order 1/(Tgov*s+1))
%--------------------------------------------------------------------------
xsg = STATE(1,:);
%--------------------------------------------------------------------------
% Turbine (second order (Ttb1*Ttb2*s + 1)/(Ttb1*Ttb2*s + (Ttb1+Ttb2)*s + 1))
%--------------------------------------------------------------------------
xt1 = STATE(2,:);
xt2 = STATE(3,:);
%--------------------------------------------------------------------------
% Grid frequency [pu]
%--------------------------------------------------------------------------
w = STATE(4,:);
%--------------------------------------------------------------------------
% Line current [pu]
%--------------------------------------------------------------------------
ir = STATE(5,:);
ii = STATE(6,:);
i = ir + 1j*ii;
%--------------------------------------------------------------------------
% Node 1 Voltage [pu]
%--------------------------------------------------------------------------
v1r = STATE(7,:);
v1i = STATE(8,:);
v1 = v1r + 1j*v1i;

%--------------------------------------------------------------------------
%% INPUT
%--------------------------------------------------------------------------
% INPUT = [in1r ; in1i]
in1r = sum(INPUT(0*nDFIG + (1:nDFIG)));
in1i = sum(INPUT(1*nDFIG + (1:nDFIG)));
%--------------------------------------------------------------------------
% Input current into node 1 [pu]
%--------------------------------------------------------------------------
MODEL.LINE.INPUT.in1_r = in1r;
MODEL.LINE.INPUT.in1_i = in1i;
in1 = in1r + 1j*in1i;
%--------------------------------------------------------------------------
% Grid voltage [pu]
%--------------------------------------------------------------------------
vgr = MODEL.GRID.INPUT.v_grid_r;
vgi = MODEL.GRID.INPUT.v_grid_i;
vg = vgr + 1j*vgi;
%--------------------------------------------------------------------------
% Grid active power reference [pu]
%--------------------------------------------------------------------------
Pg_ref = MODEL.GRID.INPUT.Pg_ref;
%--------------------------------------------------------------------------
% Load current perturbation routing (load_node: 1=PCC, 2=grid bus)
% Algebraic routing avoids if/else for Simulink compile-time dimension analysis
%--------------------------------------------------------------------------
ln2 = double(load_node == 2);
il1 = (MODEL.LINE.INPUT.il1_r + 1j*MODEL.LINE.INPUT.il1_i + ...
       (1-ln2) .* (il_r_IN + 1j*il_i_IN)) .* exp(1j*angle(v1));
il2_pert = ln2 .* (il_r_IN + 1j*il_i_IN) .* exp(1j*angle(vg));
%--------------------------------------------------------------------------
% Grid active power
%--------------------------------------------------------------------------
Pg = -real(vg.*conj(i))/sqrt(3); % Flows from the grid

%--------------------------------------------------------------------------
%% STATE DERIVATIVE
%--------------------------------------------------------------------------
%--------------------------------------------------------------------------
% Speed governor
%--------------------------------------------------------------------------
% Speed governor (first order 1/(Tgov*s+1) -> Tgov*dy + y = u
dxsg = 1./Tgov.*(-xsg + Pg_ref - 0.5*Deq_pu*(w-1));
%--------------------------------------------------------------------------
% Turbine
%--------------------------------------------------------------------------
% Second order (Ttb1*Ttb2*s + 1)/(Ttb1*Ttb2*s + (Ttb1+Ttb2)*s + 1)
% Ttb1*Ttb2*d2y + (Ttb1+Ttb2)*dy + y = Ttb1*Ttb2*du + u
% y = Ttb1*Ttb2*dz + z
% Ttb1*Ttb2*d2z + (Ttb1+Ttb2)*dz + z = u
% xt1 = z 
% xt2 = dz = dxt1
% dxt2 = d2z = 1/Ttb1/Ttb2*(-(Ttb1+Ttb2)*dz - z + u)
dxt1 = xt2;
dxt2 = 1./Ttb1./Ttb2.*(-(Ttb1+Ttb2).*xt2 - xt1 + xsg);
% Mechanical power
Pm = (Ttb1+Ttb2)*xt2 + xt1;
%--------------------------------------------------------------------------
% Frequency dynamics
%--------------------------------------------------------------------------
% Frequency
dw = 1/2/H.*(Pm - Pg*MODEL.BASE.Sb/MODEL.GRID.BASE.Sb - 0.5*Deq_pu*(w-1));
%--------------------------------------------------------------------------
% Line current [pu]
%--------------------------------------------------------------------------
di = w0.*(1./Lg.*(v1 - vg - Rg.*(i + il2_pert)) - 1j*w*i);
%--------------------------------------------------------------------------
% Node 1 Voltage [pu]
%--------------------------------------------------------------------------
dv1 = w0.*(1./Cn1.*(in1 - i - il1 - v1./Rn1) - 1j*w*v1);

%--------------------------------------------------------------------------
% State derivative
%--------------------------------------------------------------------------
STATE_DERIVATIVE = [dxsg ; dxt1 ; dxt2 ; dw ; real(di) ; imag(di) ; real(dv1) ; imag(dv1)];

%--------------------------------------------------------------------------
%% OUTPUT AND MEASURED VARIABLES
%--------------------------------------------------------------------------
% Node 1 voltage
%--------------------------------------------------------------------------
MODEL.LINE.OUTPUT.vn1_r = v1r(1);
MODEL.LINE.OUTPUT.vn1_i = v1i(1);
% PCC voltage [pu]
MODEL.LINE.OUTPUT.Vpcc = abs(v1r(1) + 1j*v1i(1));
Vpcc_OUT = MODEL.LINE.OUTPUT.Vpcc;
%--------------------------------------------------------------------------
% Node 2 voltage
%--------------------------------------------------------------------------
MODEL.LINE.OUTPUT.vn2_r = real(vg);
MODEL.LINE.OUTPUT.vn2_i = imag(vg);
%--------------------------------------------------------------------------
% Line current (from the line and into the grid)
%--------------------------------------------------------------------------
MODEL.LINE.OUTPUT.i_r = real(i);
MODEL.LINE.OUTPUT.i_i = imag(i);
%--------------------------------------------------------------------------
% Mechanical power [pu]
%--------------------------------------------------------------------------
MODEL.GRID.OUTPUT.Pmech = Pm;
%--------------------------------------------------------------------------
% Grid active power from the grid and into the line [pu] 
%--------------------------------------------------------------------------
MODEL.GRID.OUTPUT.Pgrid = Pg*MODEL.BASE.Sb/MODEL.GRID.BASE.Sb;
%--------------------------------------------------------------------------
% Grid reactive power from the grid and into the line [pu] 
%--------------------------------------------------------------------------
MODEL.GRID.OUTPUT.Qgrid = -imag(vg.*conj(i))./sqrt(3)*MODEL.BASE.Sb/MODEL.GRID.BASE.Sb;
%--------------------------------------------------------------------------
% Frequency [pu]
%--------------------------------------------------------------------------
MODEL.GRID.OUTPUT.f_pu = w;
f_OUT = MODEL.GRID.OUTPUT.f_pu;

%--------------------------------------------------------------------------
%% STATE UPDATE
%--------------------------------------------------------------------------
MODEL.GRID.STATE = STATE(1:4,:);
MODEL.LINE.STATE(1:4,:) = STATE(5:8,:);

%--------------------------------------------------------------------------
%% CONNECTIONS WITH THE POWER SYSTEM
%-------------------------------------------------------------------------
%--------------------------------------------------------------------------
% OUTPUT = [ w; v1r ; v1i]
%--------------------------------------------------------------------------
OUTPUT = zeros(3,1);
OUTPUT(1) = w;
OUTPUT(2) = v1r(1);
OUTPUT(3) = v1i(1);

return
